simulink model "a1_quad_control_thrust"  (R2018b)
settings: Solver=VariableStepAuto  StartTime=0.0  StopTime=1000  RelTol=1e-3
undefined symbols (not defined in the file or in its folder): drawQuad
libraries: simulink x4
settings Model: Creator=erics  LastModifiedBy=erics

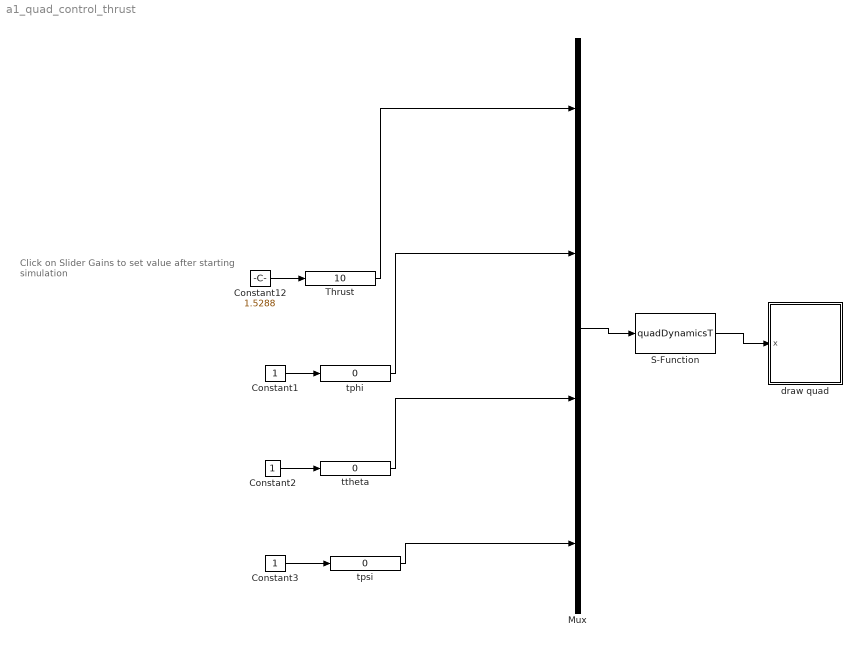
== system a1_quad_control_thrust ==
  note: Click on Slider Gains to set value
      | after starting simulation
  Constant1 : Constant
  Constant12 : Constant  Value=1.5288
  Constant2 : Constant
  Constant3 : Constant
  Mux : Mux
  S-Function : S-Function  FunctionName=quadDynamicsT  Parameters=P  SFunctionDeploymentMode=off  EnableBusSupport=off
  Thrust : simulink/Math Operations/Slider Gain  gain=10  low=-10  high=10
  draw quad : Subsystem
      mask init:
      | P.courselength = 11;
      | P.coursewidth = 6;
      |     %6ft columns plus four feet of head room
      | P.courseheight = 10;
      | 
      | % quadrotor starting point at 3 ft high and 3 ft in front of the pillars 
      | P.zstart = 0;
      | P.xstart = 0;
      | P.ystart = 0;
      | 
      | % quadrotor dimentions
      |     %2 inches from the center
      | P.boxlength = 1/6;
      | P.boxwidth = P.boxlength;
      |     %4.5 inches from the bottom to the top
      | P.boxheight = 0.375;
      |     %6 inches from box to motor
      | P.armlength = 0.5;
      |     %1/8 inch from center to the side of a rod
      | P.armwidth = 1/96;
      |     %1/4 inch from the top of the box
      | P.armposition = 1/48;
      |     %25*(2)^(1/2)/2 inches from center to perimeter along x and y axis
      | P.perimeter = 1.47;
      |     %perimeter has 3/16 inch width
      | P.periwidth = 1/64;
      | 
      | % pillar dimentions
      |     %6 ft high
      | P.pillarheight = 6;
      |     %5 ft offset;
      | P.pillarposition = 5; 
      |     %5 in radius
      | P.pillarradius = 0.417;
      |     %The adjustment for the none circular pillar
      | P.pillaradd = 0.167;
      |     %The height of each strip on color
      | P.pillarc1 = 0.833; 
      | P.pillarc2 = 0.5;
      mask Display: image(imread('tv.jpg'))
  tphi : simulink/Math Operations/Slider Gain  gain=0  low=-10  high=10
  tpsi : simulink/Math Operations/Slider Gain  gain=0  low=-10  high=10
  ttheta : simulink/Math Operations/Slider Gain  gain=0  low=-10  high=10
  wires:
  Thrust/1 -> Mux/1
  Constant2/1 -> ttheta/1
  ttheta/1 -> Mux/3
  tphi/1 -> Mux/2
  tpsi/1 -> Mux/4
  Constant1/1 -> tphi/1
  S-Function/1 -> draw quad/1(x)
  Constant12/1 -> Thrust/1
  Constant3/1 -> tpsi/1
  Mux/1 -> S-Function/1

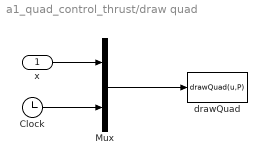
== system a1_quad_control_thrust/draw quad ==
  x : Inport
  Clock : Clock
  Mux : Mux  Inputs=2
  drawQuad : MATLABFcn  MATLABFcn=drawQuad(u,P)  OutputDimensions=0  SampleTime=0.1
  wires:
  Mux/1 -> drawQuad/1
  x/1 -> Mux/1
  Clock/1 -> Mux/2
